simulink model "FilterEq"  (R2019b)
settings: Solver=FixedStepAuto  StartTime=0.0  StopTime=10.0  FixedStep=0.2  RelTol=1e-3
settings Model: Creator=ip  LastModifiedBy=ip
settings DataIOCC: SaveOutput=off  SaveTime=off

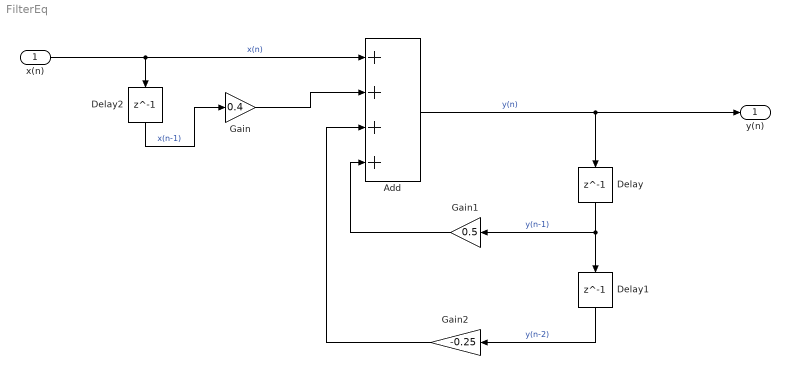
== system FilterEq ==
  x(n) : Inport  OutDataTypeStr=double  PortDimensions=1  SampleTime=[0.20000000000000001,0]
  Add : Sum  Inputs=4
  Delay : Delay  DelayLength=1
  Delay1 : Delay  DelayLength=1
  Delay2 : Delay  DelayLength=1
  Gain : Gain  Gain=0.4
  Gain1 : Gain  Gain=0.5
  Gain2 : Gain  Gain=-0.25
  y(n) : Outport  OutDataTypeStr=double  PortDimensions=1  SampleTime=[0.20000000000000001,0]
  wires:
  Gain2/1 -> Add/3
  Delay2/1 -> Gain/1  "x(n-1)"
  Delay/1 -> Delay1/1, Gain1/1  "y(n-1)"
  Gain/1 -> Add/2
  Delay1/1 -> Gain2/1  "y(n-2)"
  Gain1/1 -> Add/4
  Add/1 -> Delay/1, y(n)/1  "y(n)"
  x(n)/1 -> Delay2/1, Add/1  "x(n)"
